simulink model "Selector"  (R2020a)
settings: Solver=VariableStepAuto  StartTime=0.0  StopTime=10.0  RelTol=1e-3
values from neighbouring files (symbols this model uses):
  Eqlut = zeros(slotsAngle, slotsSpeed, 2)    [LUTScript.m]    (also in Lutscript.m = zeros(10,13,2); generateLUTs.m)
  Klut = zeros(slotsAngle, slotsSpeed, 2)    [LUTScript.m]    (also in Lutscript.m = zeros(10,13,2); generateLUTs.m)
settings Model: Creator=filip  LastModifiedBy=filip

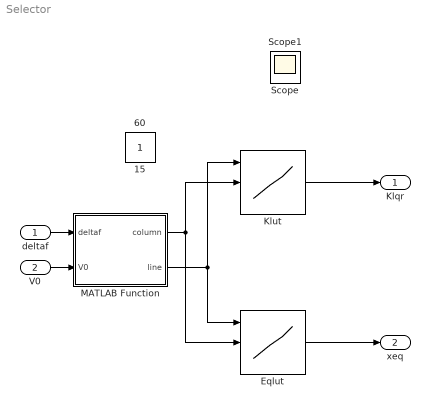
== system Selector ==
  deltaf : Inport
  V0 : Inport  Port=2
  Eqlut : Lookup_n-D  NumberOfTableDimensions=3  BreakpointsForDimension1=[1,2,3,4,5,6,7,8,9,10]  BreakpointsForDimension2=[1,2,3,4,5,6,7,8,9,10,11,12,13]  BreakpointsForDimension3=[1,2]  Table=Eqlut  InternalRulePriority=Speed  RndMeth=Simplest  InputSameDT=on
  Klut : Lookup_n-D  NumberOfTableDimensions=3  BreakpointsForDimension1=[1,2,3,4,5,6,7,8,9,10]  BreakpointsForDimension2=[1,2,3,4,5,6,7,8,9,10,11,12,13]  BreakpointsForDimension3=[1,2]  Table=Klut  InternalRulePriority=Speed  RndMeth=Simplest  InputSameDT=on
  MATLAB Function : MATLAB Function  TreatAsAtomicUnit=on
  Klqr : Outport
  xeq : Outport  Port=2
  15 : Constant  IOType=siggen
  60 : Constant  IOType=siggen
  Scope : Scope
  Scope1 : Scope
  wires:
  MATLAB Function/1(column) -> Klut/2, Eqlut/2
  MATLAB Function/2(line) -> Eqlut/1, Klut/1
  deltaf/1 -> MATLAB Function/1(deltaf)
  V0/1 -> MATLAB Function/2(V0)
  Klut/1 -> Klqr/1
  Eqlut/1 -> xeq/1

== matlab function Selector/MATLAB Function ==
  data: deltaf input; column output; V0 input; line output
function [column, line]= Selector(deltaf, V0)
column = round(V0/10);
line = (round(deltaf/3));
